simulink model "Rektifikaciya_AVO"  (Simulink 7.5)
settings: Solver=ode23tb  StartTime=0.0  StopTime=400000  FixedStep=0.1  RelTol=1e-3
libraries: simulink x2
settings Model: Creator=User  LastModifiedBy=Mithra
settings OptimizationCC: InitFltsAndDblsToZero=on
settings DebuggingCC: StrictBusMsg=Warning

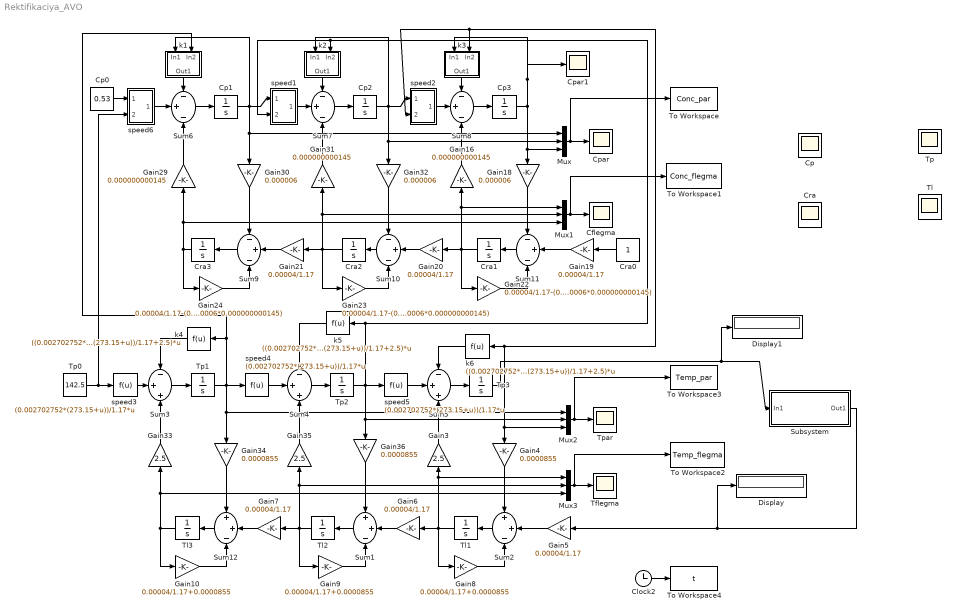
== system Rektifikaciya_AVO ==
  Cflegma : Scope
      settings: SaveName=ScopeData5
  Clock2 : Clock
      settings: Decimation=10
  Cp : Scope  NumInputPorts=3
      settings: TimeRange=12  YMin=61.5~77~95.34999999999999  YMax=62.5~82~95.37000000000001
  Cp0 : Constant  Value=0.53
  Cp1 : Integrator  InitialCondition=0.665
  Cp2 : Integrator  InitialCondition=0.803
  Cp3 : Integrator  InitialCondition=0.986
  Cpar : Scope
      settings: SaveName=ScopeData4
  Cpar1 : Scope
      settings: SaveName=ScopeData10
  Cra : Scope  NumInputPorts=3
      settings: YMin=4.17~2.4~0.84  YMax=4.28~2.5~1
  Cra0 : Constant
  Cra1 : Integrator  InitialCondition=0.827
  Cra2 : Integrator  InitialCondition=0.6862
  Cra3 : Integrator  InitialCondition=0.5696
  Display : Display
  Display1 : Display
  Gain10 : Gain  Gain=0.00004/1.17+0.0000855
  Gain16 : Gain  Gain=0.000000000145
  Gain18 : Gain  Gain=0.000006
  Gain{5..7,19..21} (6 alike) : Gain  Gain=0.00004/1.17
  Gain22 : Gain  Gain=0.00004/1.17-(0.000006*0.000000000145)
  Gain23 : Gain  Gain=0.00004/1.17-(0.000006*0.000000000145)
  Gain24 : Gain  Gain=0.00004/1.17-(0.000006*0.000000000145)
  Gain29 : Gain  Gain=0.000000000145
  Gain3 : Gain  Gain=2.5
  Gain30 : Gain  Gain=0.000006
  Gain31 : Gain  Gain=0.000000000145
  Gain32 : Gain  Gain=0.000006
  Gain33 : Gain  Gain=2.5
  Gain34 : Gain  Gain=0.0000855
  Gain35 : Gain  Gain=2.5
  Gain36 : Gain  Gain=0.0000855
  Gain4 : Gain  Gain=0.0000855
  Gain8 : Gain  Gain=0.00004/1.17+0.0000855
  Gain9 : Gain  Gain=0.00004/1.17+0.0000855
  Mux{,1..3} (4 alike) : Mux  Inputs=3
  Subsystem : Subsystem
  Sum1 : Sum  Inputs=++-
  Sum{6..11} (6 alike) : Sum  Inputs=-+-
  Sum12 : Sum  Inputs=++-
  Sum2 : Sum  Inputs=++-
  Sum3 : Sum  Inputs=-++
  Sum4 : Sum  Inputs=-++
  Sum5 : Sum  Inputs=-++
  Tflegma : Scope
      settings: SaveName=ScopeData7
  Tl : Scope  NumInputPorts=3
      settings: YMin=13~10~8.800000000000001  YMax=15.2~21~10.55  SaveName=ScopeData3
  Tl1 : Integrator  InitialCondition=58.28
  Tl2 : Integrator  InitialCondition=86.23
  Tl3 : Integrator  InitialCondition=111.75
  To Workspace : ToWorkspace  VariableName=Conc_par  SampleTime=-1  SaveFormat=Array
  To Workspace1 : ToWorkspace  VariableName=Conc_flegma  SampleTime=-1  SaveFormat=Array
  To Workspace2 : ToWorkspace  VariableName=Temp_flegma  SampleTime=-1  SaveFormat=Array
  To Workspace3 : ToWorkspace  VariableName=Temp_par  SampleTime=-1  SaveFormat=Array
  To Workspace4 : ToWorkspace  VariableName=t  SampleTime=-1  SaveFormat=Array
  Tp : Scope  NumInputPorts=3
      settings: TimeRange=12  YMin=155.5~145~146  YMax=158.5~152~154.5  SaveName=ScopeData2
  Tp0 : Constant  Value=142.5
  Tp1 : Integrator  InitialCondition=121.956
  Tp2 : Integrator  InitialCondition=97.4
  Tp3 : Integrator  InitialCondition=69.6  IgnoreLimit=on
  Tpar : Scope
      settings: SaveName=ScopeData6
  k1 : Subsystem
  k2 : Subsystem
  k3 : Subsystem
  k4 : Fcn  Expr=((0.002702752*(273.15+u))/1.17+2.5)*u
  k5 : Fcn  Expr=((0.002702752*(273.15+u))/1.17+2.5)*u
  k6 : Fcn  Expr=((0.002702752*(273.15+u))/1.17+2.5)*u
  speed1 : Subsystem
  speed2 : Subsystem
  speed3 : Fcn  Expr=(0.002702752*(273.15+u))/1.17*u
  speed4 : Fcn  Expr=(0.002702752*(273.15+u))/1.17*u
  speed5 : Fcn  Expr=(0.002702752*(273.15+u))/1.17*u
  speed6 : Subsystem
  wires:
  Sum6/1 -> Cp1/1
  speed1/1(Out1) -> Sum7/2
  Sum7/1 -> Cp2/1
  speed2/1(Out1) -> Sum8/2
  Sum8/1 -> Cp3/1
  Cp1/1 -> Gain30/1, Mux/1, speed1/1(In1), k1/1(In1)
  Cp2/1 -> Gain32/1, Mux/2, speed2/1(In1), k2/1(In1)
  Gain29/1 -> Sum6/3
  Cp3/1 -> Gain18/1, Mux/3, k3/1(In1), Cpar1/1
  Gain31/1 -> Sum7/3
  Gain16/1 -> Sum8/3
  Gain30/1 -> Sum9/1
  Gain32/1 -> Sum10/1
  Gain18/1 -> Sum11/1
  Gain19/1 -> Sum11/2
  Sum11/1 -> Cra1/1
  Cra1/1 -> Gain22/1, Gain20/1, Gain16/1, Mux1/1
  Gain20/1 -> Sum10/2
  Sum10/1 -> Cra2/1
  Cra2/1 -> Gain23/1, Gain21/1, Gain31/1, Mux1/2
  Gain21/1 -> Sum9/2
  Sum9/1 -> Cra3/1
  Cra3/1 -> Gain24/1, Gain29/1, Mux1/3
  Gain22/1 -> Sum11/3
  Gain23/1 -> Sum10/3
  Gain24/1 -> Sum9/3
  speed3/1 -> Sum3/2
  k4/1 -> Sum3/1
  Sum3/1 -> Tp1/1
  speed4/1 -> Sum4/2
  k5/1 -> Sum4/1
  Sum4/1 -> Tp2/1
  speed5/1 -> Sum5/2
  k6/1 -> Sum5/1
  Sum5/1 -> Tp3/1
  Tp1/1 -> Gain34/1, Mux2/1, k4/1, k1/2(In2), speed4/1
  Tp2/1 -> Gain36/1, Mux2/2, k5/1, speed1/2(In2), k2/2(In2), speed5/1
  Gain33/1 -> Sum3/3
  Tp3/1 -> Gain4/1, Mux2/3, k6/1, k3/2(In2), speed2/2(In2), Subsystem/1(In1), Display1/1
  Gain35/1 -> Sum4/3
  Gain3/1 -> Sum5/3
  Gain34/1 -> Sum12/1
  Gain36/1 -> Sum1/1
  Gain4/1 -> Sum2/1
  Gain5/1 -> Sum2/2
  Sum2/1 -> Tl1/1
  Tl1/1 -> Gain8/1, Gain6/1, Gain3/1, Mux3/1
  Gain6/1 -> Sum1/2
  Sum1/1 -> Tl2/1
  Tl2/1 -> Gain9/1, Gain7/1, Gain35/1, Mux3/2
  Gain7/1 -> Sum12/2
  Sum12/1 -> Tl3/1
  Tl3/1 -> Gain10/1, Gain33/1, Mux3/3
  Gain8/1 -> Sum2/3
  Gain9/1 -> Sum1/3
  Gain10/1 -> Sum12/3
  Tp0/1 -> speed3/1, speed6/2(In2)
  speed6/1(Out1) -> Sum6/2
  Cp0/1 -> speed6/1(In1)
  k1/1(Out1) -> Sum6/1
  k2/1(Out1) -> Sum7/1
  k3/1(Out1) -> Sum8/1
  Cra0/1 -> Gain19/1
  Mux/1 -> Cpar/1, To Workspace/1
  Mux1/1 -> Cflegma/1, To Workspace1/1
  Mux2/1 -> Tpar/1, To Workspace3/1
  Mux3/1 -> Tflegma/1, To Workspace2/1
  Clock2/1 -> To Workspace4/1
  Subsystem/1(Out1) -> Gain5/1, Display/1

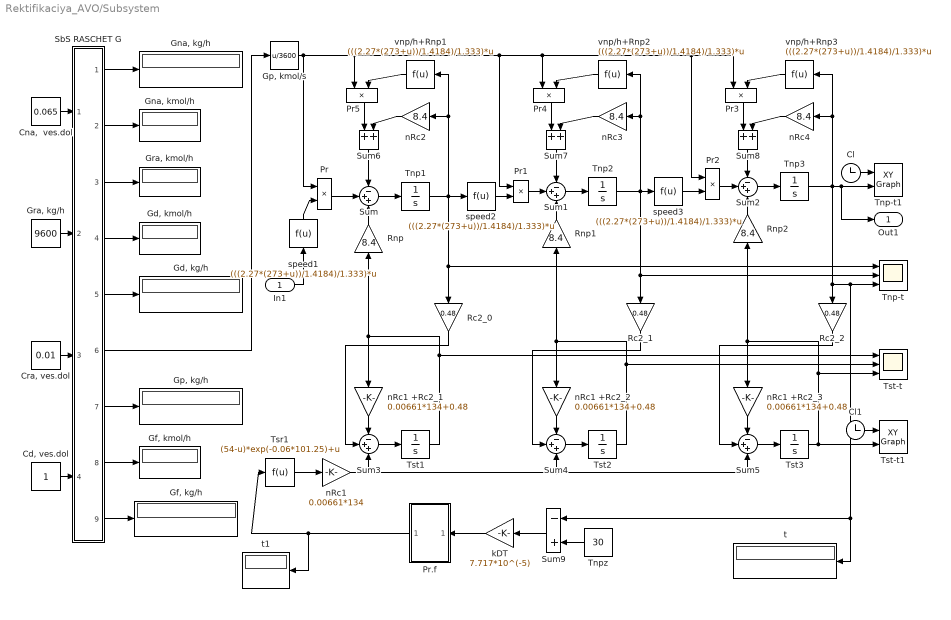
== system Rektifikaciya_AVO/Subsystem ==
  In1 : Inport  OutDataType=fixdt(1, 16)  OutScaling=2^0
  "Cd, ves.dol" : Constant
  Cl : Clock
      settings: Decimation=10
  Cl1 : Clock
      settings: Decimation=10
  "Cna,  ves.dol" : Constant  Value=0.065
  "Cra, ves.dol" : Constant  Value=0.01
  "Gd, kg/h" : Display
  "Gd, kmol/h" : Display
  "Gf, kg/h" : Display
  "Gf, kmol/h" : Display
  "Gna, kg/h" : Display
  "Gna, kmol/h" : Display
  "Gp, kmol/s" : Fcn  Expr=u/3600
  "Gp, kg/h" : Display
  "Gra, kg/h" : Constant  Value=9600
  "Gra, kmol/h" : Display
  Pr{,1..5} (6 alike) : Product  RndMeth=Zero
  Pr.f : Subsystem
  Rc2_0 : Gain  Gain=0.48
  Rc2_1 : Gain  Gain=0.48
  Rc2_2 : Gain  Gain=0.48
  Rnp : Gain  Gain=8.4
  Rnp1 : Gain  Gain=8.4
  Rnp2 : Gain  Gain=8.4
  SbS RASCHET G : Subsystem
  Sum{,1..5} (6 alike) : Sum  Inputs=-++
  Sum6 : Sum
  Sum7 : Sum
  Sum8 : Sum
  Sum9 : Sum  Inputs=-+
  Tnp-t : Scope  NumInputPorts=3
      settings: YMin=67.9728~67.0823~66.2033  YMax=75.1278~74.1435~73.1721  SaveName=ScopeData8
  Tnp-t1 : simulink/Sinks/XY Graph  SystemSampleTime=-1  xmin=0  xmax=1000  ymin=10  ymax=50  st=-1
  Tnp1 : Integrator  InitialCondition=55.042986606641151
  Tnp2 : Integrator  InitialCondition=42.494060413287038
  Tnp3 : Integrator  InitialCondition=33.818616670435347
  Tnpz : Constant  Value=30
  Tsr1 : Fcn  Expr=(54-u)*exp(-0.06*101.25)+u
  Tst-t : Scope  NumInputPorts=3
      settings: YMin=320.767~573.618~826.668  YMax=354.532~633.998~913.686  SaveName=ScopeData9
  Tst-t1 : simulink/Sinks/XY Graph  SystemSampleTime=-1  xmin=0  xmax=1000  ymin=10  ymax=50  st=-1
  Tst1 : Integrator  InitialCondition=30.749212884999000
  Tst2 : Integrator  InitialCondition=26.338794670104530
  Tst3 : Integrator  InitialCondition=23.289742144317184
  kDT : Gain  Gain=7.717*10^(-5)
  nRc1 : Gain  Gain=0.00661*134
  nRc1 +Rc2_1 : Gain  Gain=0.00661*134+0.48
  nRc1 +Rc2_2 : Gain  Gain=0.00661*134+0.48
  nRc1 +Rc2_3 : Gain  Gain=0.00661*134+0.48
  nRc2 : Gain  Gain=8.4
  nRc3 : Gain  Gain=8.4
  nRc4 : Gain  Gain=8.4
  speed1 : Fcn  Expr=(((2.27*(273+u))/1.4184)/1.333)*u
  speed2 : Fcn  Expr=(((2.27*(273+u))/1.4184)/1.333)*u
  speed3 : Fcn  Expr=(((2.27*(273+u))/1.4184)/1.333)*u
  t : Display
  t1 : Display
  vnp/h+Rnp1 : Fcn  Expr=(((2.27*(273+u))/1.4184)/1.333)*u
  vnp/h+Rnp2 : Fcn  Expr=(((2.27*(273+u))/1.4184)/1.333)*u
  vnp/h+Rnp3 : Fcn  Expr=(((2.27*(273+u))/1.4184)/1.333)*u
  Out1 : Outport  OutDataType=fixdt(1, 16)  OutScaling=2^0
  wires:
  Sum/1 -> Tnp1/1
  Tnp1/1 -> speed2/1, Rc2_0/1, Tnp-t/1, vnp/h+Rnp1/1, nRc2/1
  Sum1/1 -> Tnp2/1
  Tnp2/1 -> speed3/1, Rc2_1/1, Tnp-t/2, vnp/h+Rnp2/1, nRc3/1
  Sum2/1 -> Tnp3/1
  Tnp3/1 -> vnp/h+Rnp3/1, nRc4/1, Tnp-t1/2, Out1/1, Rc2_2/1, Tnp-t/3, t/1, Sum9/1
  Cl/1 -> Tnp-t1/1
  Rnp1/1 -> Sum1/3
  Rnp2/1 -> Sum2/3
  nRc1 +Rc2_1/1 -> Sum3/1
  Sum3/1 -> Tst1/1
  nRc1 +Rc2_2/1 -> Sum4/1
  Sum4/1 -> Tst2/1
  Tst2/1 -> nRc1 +Rc2_2/1, Rnp1/1, Tst-t/2
  nRc1 +Rc2_3/1 -> Sum5/1
  Sum5/1 -> Tst3/1
  nRc1/1 -> Sum3/3, Sum5/3, Sum4/3
  Rnp/1 -> Sum/3
  Tst1/1 -> nRc1 +Rc2_1/1, Rnp/1, Tst-t/1
  Tst3/1 -> Tst-t1/2, nRc1 +Rc2_3/1, Rnp2/1, Tst-t/3
  Rc2_1/1 -> Sum4/2
  Rc2_2/1 -> Sum5/2
  Rc2_0/1 -> Sum3/2
  Cl1/1 -> Tst-t1/1
  speed1/1 -> Pr/2
  "Gp, kmol/s"/1 -> Pr/1, Pr5/1, Pr2/1, Pr3/1, Pr4/1, Pr1/1
  Pr/1 -> Sum/2
  Pr1/1 -> Sum1/2
  speed2/1 -> Pr1/2
  Pr2/1 -> Sum2/2
  speed3/1 -> Pr2/2
  vnp/h+Rnp3/1 -> Pr3/2
  vnp/h+Rnp2/1 -> Pr4/2
  vnp/h+Rnp1/1 -> Pr5/2
  Pr5/1 -> Sum6/1
  Sum6/1 -> Sum/1
  nRc2/1 -> Sum6/2
  nRc3/1 -> Sum7/2
  Pr4/1 -> Sum7/1
  Sum7/1 -> Sum1/1
  nRc4/1 -> Sum8/2
  Pr3/1 -> Sum8/1
  Sum8/1 -> Sum2/1
  "Cna,  ves.dol"/1 -> SbS RASCHET G/1(In1)
  "Cra, ves.dol"/1 -> SbS RASCHET G/3(In3)
  "Cd, ves.dol"/1 -> SbS RASCHET G/4(In4)
  "Gra, kg/h"/1 -> SbS RASCHET G/2(In2)
  SbS RASCHET G/1(Out1) -> "Gna, kg/h"/1
  SbS RASCHET G/5(Out5) -> "Gd, kg/h"/1
  SbS RASCHET G/7(Out7) -> "Gp, kg/h"/1
  SbS RASCHET G/9(Out9) -> "Gf, kg/h"/1
  SbS RASCHET G/2(Out2) -> "Gna, kmol/h"/1
  SbS RASCHET G/3(Out3) -> "Gra, kmol/h"/1
  SbS RASCHET G/4(Out4) -> "Gd, kmol/h"/1
  SbS RASCHET G/6(Out6) -> "Gp, kmol/s"/1
  SbS RASCHET G/8(Out8) -> "Gf, kmol/h"/1
  In1/1 -> speed1/1
  Sum9/1 -> kDT/1
  Tnpz/1 -> Sum9/2
  Pr.f/1(Out1) -> t1/1, Tsr1/1
  kDT/1 -> Pr.f/1(In1)
  Tsr1/1 -> nRc1/1

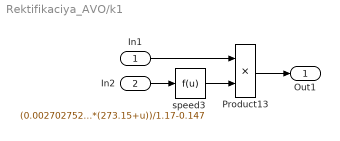
== system Rektifikaciya_AVO/k1 ==
  In1 : Inport
  In2 : Inport  Port=2
  Product13 : Product  SaturateOnIntegerOverflow=on  InputSameDT=on  OutDataTypeStr=Inherit: Same as first input
  speed3 : Fcn  Expr=(0.002702752*(273.15+u))/1.17-0.147
  Out1 : Outport
  wires:
  Product13/1 -> Out1/1
  speed3/1 -> Product13/2
  In2/1 -> speed3/1
  In1/1 -> Product13/1

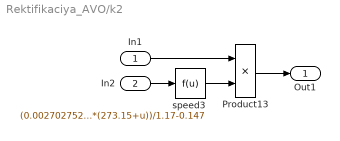
== system Rektifikaciya_AVO/k2 ==
  In1 : Inport
  In2 : Inport  Port=2
  Product13 : Product  SaturateOnIntegerOverflow=on  InputSameDT=on  OutDataTypeStr=Inherit: Same as first input
  speed3 : Fcn  Expr=(0.002702752*(273.15+u))/1.17-0.147
  Out1 : Outport
  wires:
  In1/1 -> Product13/1
  In2/1 -> speed3/1
  speed3/1 -> Product13/2
  Product13/1 -> Out1/1

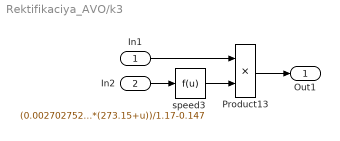
== system Rektifikaciya_AVO/k3 ==
  In1 : Inport
  In2 : Inport  Port=2
  Product13 : Product  SaturateOnIntegerOverflow=on  InputSameDT=on  OutDataTypeStr=Inherit: Same as first input
  speed3 : Fcn  Expr=(0.002702752*(273.15+u))/1.17-0.147
  Out1 : Outport
  wires:
  Product13/1 -> Out1/1
  speed3/1 -> Product13/2
  In2/1 -> speed3/1
  In1/1 -> Product13/1

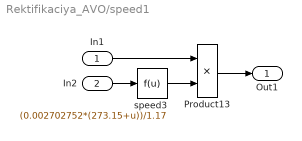
== system Rektifikaciya_AVO/speed1 ==
  In1 : Inport
  In2 : Inport  Port=2
  Product13 : Product  SaturateOnIntegerOverflow=on  InputSameDT=on  OutDataTypeStr=Inherit: Same as first input
  speed3 : Fcn  Expr=(0.002702752*(273.15+u))/1.17
  Out1 : Outport
  wires:
  Product13/1 -> Out1/1
  speed3/1 -> Product13/2
  In2/1 -> speed3/1
  In1/1 -> Product13/1

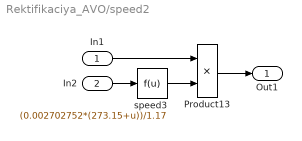
== system Rektifikaciya_AVO/speed2 ==
  In1 : Inport
  In2 : Inport  Port=2
  Product13 : Product  SaturateOnIntegerOverflow=on  InputSameDT=on  OutDataTypeStr=Inherit: Same as first input
  speed3 : Fcn  Expr=(0.002702752*(273.15+u))/1.17
  Out1 : Outport
  wires:
  In1/1 -> Product13/1
  In2/1 -> speed3/1
  speed3/1 -> Product13/2
  Product13/1 -> Out1/1

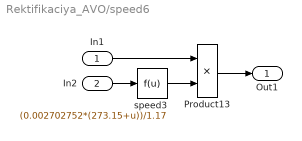
== system Rektifikaciya_AVO/speed6 ==
  In1 : Inport
  In2 : Inport  Port=2
  Product13 : Product  SaturateOnIntegerOverflow=on  InputSameDT=on  OutDataTypeStr=Inherit: Same as first input
  speed3 : Fcn  Expr=(0.002702752*(273.15+u))/1.17
  Out1 : Outport
  wires:
  In1/1 -> Product13/1
  In2/1 -> speed3/1
  speed3/1 -> Product13/2
  Product13/1 -> Out1/1

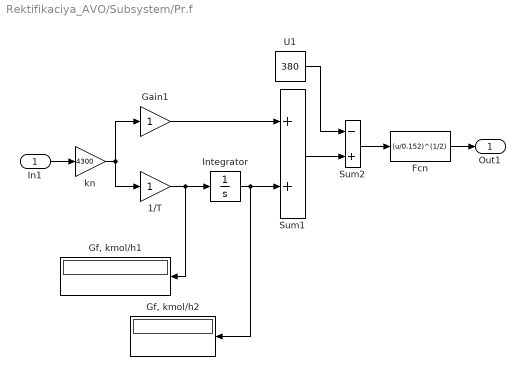
== system Rektifikaciya_AVO/Subsystem/Pr.f ==
  In1 : Inport
  1/T : Gain
  Fcn : Fcn  Expr=(u/0.152)^(1/2)
  Gain1 : Gain
  "Gf, kmol/h1" : Display
  "Gf, kmol/h2" : Display
  Integrator : Integrator  InitialCondition=403.6
  Sum1 : Sum
  Sum2 : Sum  Inputs=-+
  U1 : Constant  Value=380
  kn : Gain  Gain=4300
  Out1 : Outport
  wires:
  kn/1 -> 1/T/1, Gain1/1
  1/T/1 -> Integrator/1, "Gf, kmol/h1"/1
  Integrator/1 -> Sum1/2, "Gf, kmol/h2"/1
  Gain1/1 -> Sum1/1
  Sum1/1 -> Sum2/2
  U1/1 -> Sum2/1
  In1/1 -> kn/1
  Fcn/1 -> Out1/1
  Sum2/1 -> Fcn/1

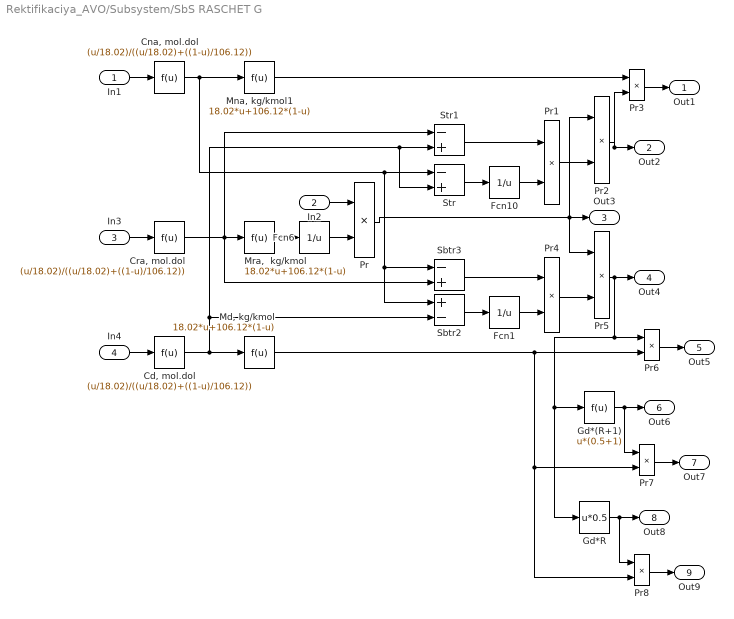
== system Rektifikaciya_AVO/Subsystem/SbS RASCHET G ==
  In1 : Inport
  In2 : Inport  Port=2
  In3 : Inport  Port=3
  In4 : Inport  Port=4
  "Cd, mol.dol" : Fcn  Expr=(u/18.02)/((u/18.02)+((1-u)/106.12))
  "Cna, mol.dol" : Fcn  Expr=(u/18.02)/((u/18.02)+((1-u)/106.12))
  "Cra, mol.dol" : Fcn  Expr=(u/18.02)/((u/18.02)+((1-u)/106.12))
  Fcn1 : Fcn  Expr=1/u
  Fcn10 : Fcn  Expr=1/u
  Fcn6 : Fcn  Expr=1/u
  Gd*(R+1) : Fcn  Expr=u*(0.5+1)
  Gd*R : Fcn  Expr=u*0.5
  "Md, kg/kmol" : Fcn  Expr=18.02*u+106.12*(1-u)
  "Mna, kg/kmol1" : Fcn  Expr=18.02*u+106.12*(1-u)
  "Mra,  kg/kmol" : Fcn  Expr=18.02*u+106.12*(1-u)
  Pr{,1..8} (9 alike) : Product  RndMeth=Zero
  Sbtr2 : Sum  Inputs=+-
  Sbtr3 : Sum  Inputs=-+
  Str : Sum  Inputs=-+
  Str1 : Sum  Inputs=-+
  Out1 : Outport
  Out2 : Outport  Port=2
  Out3 : Outport  Port=3
  Out4 : Outport  Port=4
  Out5 : Outport  Port=5
  Out6 : Outport  Port=6
  Out7 : Outport  Port=7
  Out8 : Outport  Port=8
  Out9 : Outport  Port=9
  wires:
  "Mna, kg/kmol1"/1 -> Pr3/1
  "Cna, mol.dol"/1 -> "Mna, kg/kmol1"/1, Str/1, Sbtr3/1, Sbtr2/1
  "Cra, mol.dol"/1 -> "Mra,  kg/kmol"/1, Str1/1, Sbtr3/2
  "Cd, mol.dol"/1 -> "Md, kg/kmol"/1, Str1/2, Str/2, Sbtr2/2
  "Mra,  kg/kmol"/1 -> Fcn6/1
  Fcn6/1 -> Pr/2
  Pr/1 -> Pr2/1, Out3/1, Pr5/1
  Str/1 -> Fcn10/1
  Fcn10/1 -> Pr1/2
  Pr2/1 -> Pr3/2, Out2/1
  Pr1/1 -> Pr2/2
  Str1/1 -> Pr1/1
  Fcn1/1 -> Pr4/2
  Pr5/1 -> Pr6/1, Gd*(R+1)/1, Gd*R/1, Out4/1
  Pr4/1 -> Pr5/2
  "Md, kg/kmol"/1 -> Pr6/2, Pr7/2, Pr8/2
  Sbtr2/1 -> Fcn1/1
  Sbtr3/1 -> Pr4/1
  Gd*(R+1)/1 -> Pr7/1, Out6/1
  Gd*R/1 -> Pr8/1, Out8/1
  In1/1 -> "Cna, mol.dol"/1
  Pr3/1 -> Out1/1
  In2/1 -> Pr/1
  In3/1 -> "Cra, mol.dol"/1
  Pr6/1 -> Out5/1
  In4/1 -> "Cd, mol.dol"/1
  Pr7/1 -> Out7/1
  Pr8/1 -> Out9/1
